simulink model "SimulNro2_20230617"  (R2022b)
settings: Solver=ode4  StartTime=0.0  StopTime=1  FixedStep=.001  RelTol=1e-3
libraries: cstblocks x2
settings Model: Creator=aghersin  LastModifiedBy=aghersin

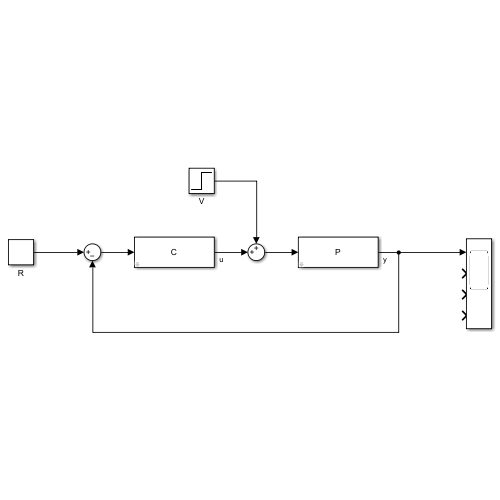
[thumbnail: Simulink's stored preview of the top-level diagram]
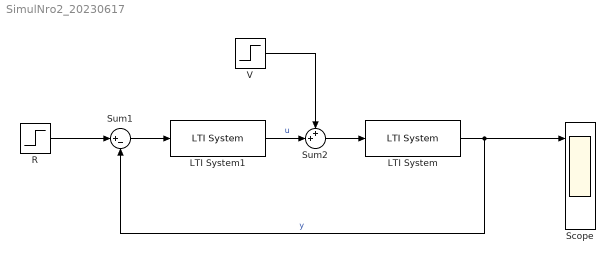
== system SimulNro2_20230617 ==
  LTI System : cstblocks/LTI System  sys=P  IC=[]
  LTI System1 : cstblocks/LTI System  sys=C  IC=[]
  R : Step  Time=.1  SampleTime=0
  Scope : Scope  NumInputPorts=4
  Sum1 : Sum  Inputs=|+-
  Sum2 : Sum  Inputs=++|
  V : Step  SampleTime=0
  wires:
  R/1 -> Sum1/1
  LTI System/1 -> Sum1/2, Scope/1  "y"
  LTI System1/1 -> Sum2/2  "u"
  Sum1/1 -> LTI System1/1
  Sum2/1 -> LTI System/1
  V/1 -> Sum2/1
